simulink subsystem "ProcNav"  (R2021a)
settings: Solver=VariableStepAuto  StartTime=0.0  StopTime=10.0  RelTol=1e-3
undefined symbols (not defined in the file): DiscIntNeverNeededParam, physics
libraries: aerolibutil x9, sharedtransform x2, sharedTrackingLibrary x1
settings Model: Creator=Lamarre  LastModifiedBy=lamarre
settings SolverCC: AlgebraicLoopSolver=TrustRegion
settings DebuggingCC: SFMachineParentedDataDiag=warning

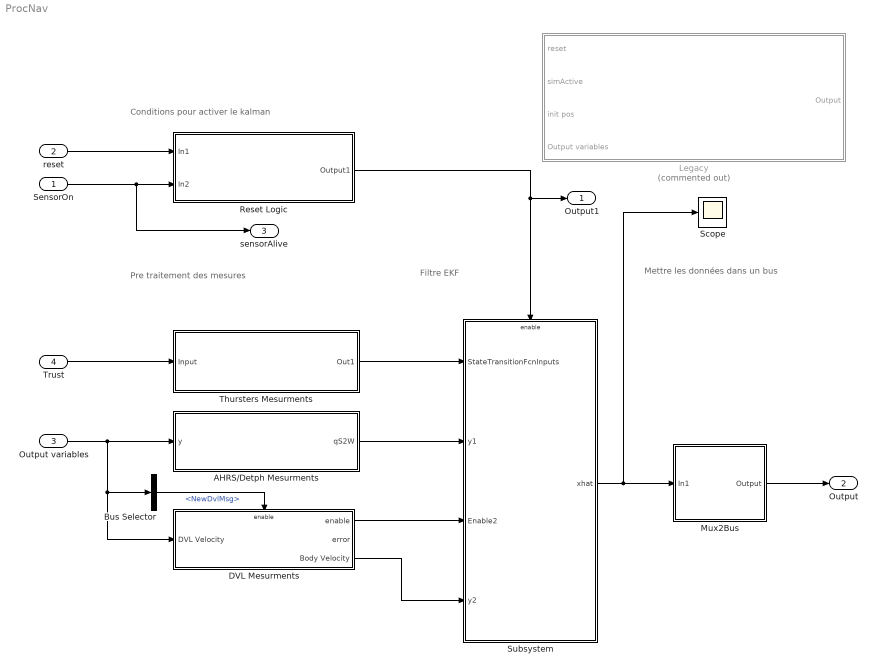
== system ProcNav ==
  note: Conditions pour activer le kalman
  note: Filtre EKF
  note: Pre traitement des mesures
  note: Mettre les données
      | dans un bus
  SensorOn : Inport
  reset : Inport  Port=2
  Output variables : Inport  Port=3
  Trust : Inport  Port=4
  AHRS/Detph Mesurments : Subsystem
  Bus Selector : BusSelector  OutputSignals=NewDvlMsg
  DVL Mesurments : Subsystem
  Legacy : Subsystem  Commented=on
  Mux2Bus : Subsystem
  Reset Logic : Subsystem
  Scope : Scope
  Subsystem : Subsystem
  Thursters Mesurments : Subsystem
  Output1 : Outport
  Output : Outport  Port=2
  sensorAlive : Outport  Port=3
  wires:
  DVL Mesurments/3(Body Velocity) -> Subsystem/4(y2)
  AHRS/Detph Mesurments/1(qS2W) -> Subsystem/2(y1)
  DVL Mesurments/1(enable) -> Subsystem/3(Enable2)
  Subsystem/1(xhat) -> Mux2Bus/1(In1), Scope/1
  Thursters Mesurments/1(Out1) -> Subsystem/1(StateTransitionFcnInputs)
  Output variables/1 -> DVL Mesurments/1(DVL Velocity), Bus Selector/1, AHRS/Detph Mesurments/1(y)
  Trust/1 -> Thursters Mesurments/1(Input)
  reset/1 -> Reset Logic/1(In1)
  SensorOn/1 -> Reset Logic/2(In2), sensorAlive/1
  Mux2Bus/1(Output) -> Output/1
  Bus Selector/1 -> DVL Mesurments/Enable  "<NewDvlMsg>"
  Reset Logic/1(Output1) -> Subsystem/Enable, Output1/1

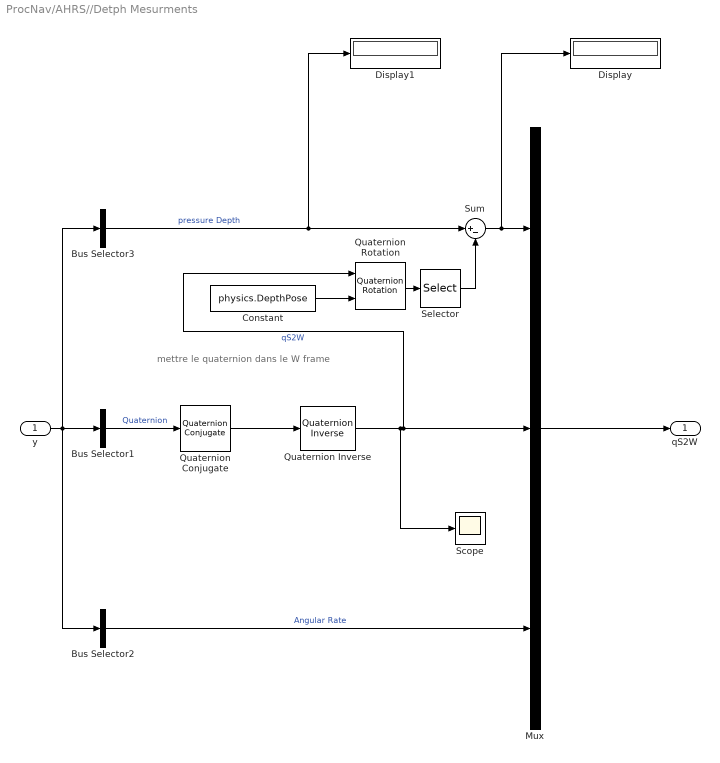
== system ProcNav/AHRS//Detph Mesurments ==
  note: mettre le quaternion dans le W frame
  y : Inport
  Bus Selector1 : BusSelector  OutputSignals=Quaternion  OutputAsBus=on
  Bus Selector2 : BusSelector  OutputSignals=Angular Rate  OutputAsBus=on
  Bus Selector3 : BusSelector  OutputSignals=Pressure Depth.Data  OutputAsBus=on
  Constant : Constant  Value=physics.DepthPose
  Display : Display
  Display1 : Display
  Mux : Mux  Inputs=3
  Quaternion Conjugate : aerolibutil/Quaternion Conjugate
      settings: SourceProductBaseCode=AE
  Quaternion Inverse : aerolibutil/Quaternion Inverse
  Quaternion Rotation : aerolibutil/Quaternion Rotation
  Scope : Scope
  Selector : Selector  InputPortWidth=3  IndexOptions=Index vector (dialog)  Indices=[3]  OutputSizes=1
  Sum : Sum  Inputs=|+-
  qS2W : Outport
  wires:
  Sum/1 -> Mux/1, Display/1
  Quaternion Rotation/1 -> Selector/1
  Selector/1 -> Sum/2
  Constant/1 -> Quaternion Rotation/2
  Bus Selector3/1 -> Sum/1, Display1/1  "pressure Depth"
  Quaternion Conjugate/1 -> Quaternion Inverse/1
  Mux/1 -> qS2W/1
  Bus Selector2/1 -> Mux/3  "Angular Rate"
  Quaternion Inverse/1 -> Mux/2, Quaternion Rotation/1, Scope/1  "qS2W"
  Bus Selector1/1 -> Quaternion Conjugate/1  "Quaternion"
  y/1 -> Bus Selector1/1, Bus Selector3/1, Bus Selector2/1

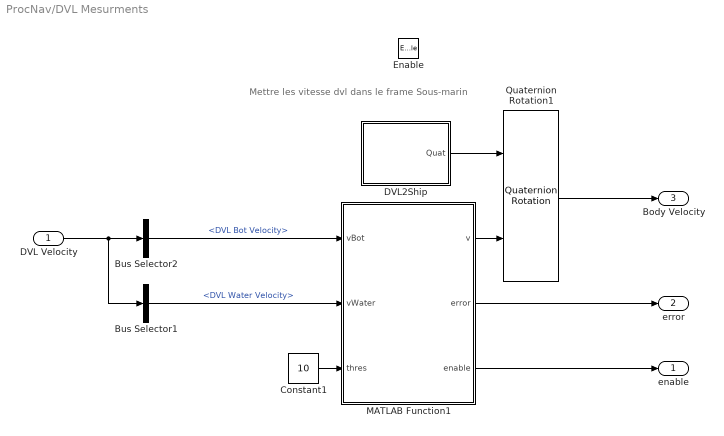
== system ProcNav/DVL Mesurments ==
  note: Mettre les vitesse dvl dans le frame Sous-marin
  DVL Velocity : Inport
  Enable : EnablePort
  Bus Selector1 : BusSelector  OutputSignals=DVL Water Velocity
  Bus Selector2 : BusSelector  OutputSignals=DVL Bot Velocity
  Constant1 : Constant  Value=10
  DVL2Ship : Subsystem
  MATLAB Function1 : MATLAB Function  TreatAsAtomicUnit=on
  Quaternion Rotation1 : aerolibutil/Quaternion Rotation
  enable : Outport
  error : Outport  Port=2
  Body Velocity : Outport  Port=3
  wires:
  MATLAB Function1/3(enable) -> enable/1
  Quaternion Rotation1/1 -> Body Velocity/1
  MATLAB Function1/2(error) -> error/1
  Bus Selector1/1 -> MATLAB Function1/2(vWater)  "<DVL Water Velocity>"
  Bus Selector2/1 -> MATLAB Function1/1(vBot)  "<DVL Bot Velocity>"
  DVL Velocity/1 -> Bus Selector2/1, Bus Selector1/1
  MATLAB Function1/1(v) -> Quaternion Rotation1/2
  Constant1/1 -> MATLAB Function1/3(thres)
  DVL2Ship/1(Quat) -> Quaternion Rotation1/1

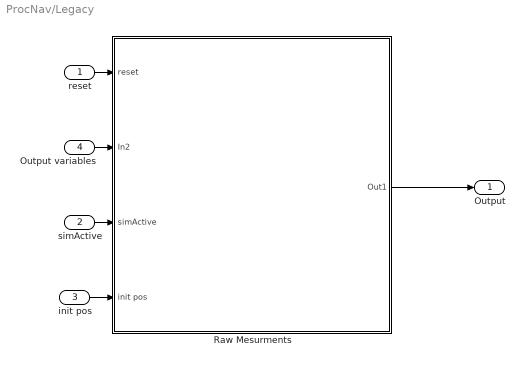
== system ProcNav/Legacy ==
  reset : Inport
  simActive : Inport  Port=2
  init pos : Inport  Port=3
  Output variables : Inport  Port=4
  "Raw Mesurments " : Subsystem
  Output : Outport
  wires:
  "Raw Mesurments "/1(Out1) -> Output/1
  init pos/1 -> "Raw Mesurments "/4(init pos)
  Output variables/1 -> "Raw Mesurments "/2(In2)
  reset/1 -> "Raw Mesurments "/1(reset)
  simActive/1 -> "Raw Mesurments "/3(simActive)

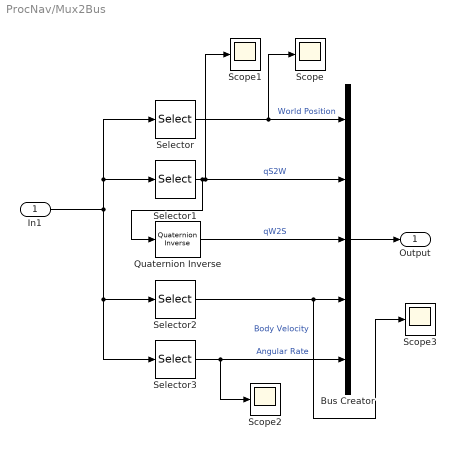
== system ProcNav/Mux2Bus ==
  In1 : Inport
  Bus Creator : BusCreator  Inputs=5
  Quaternion Inverse : aerolibutil/Quaternion Inverse
  Scope{,1..3} (4 alike) : Scope
  Selector : Selector  InputPortWidth=13  IndexOptions=Index vector (dialog)  Indices=[1:3]  OutputSizes=1
  Selector1 : Selector  InputPortWidth=13  IndexOptions=Index vector (dialog)  Indices=[4:7]  OutputSizes=1
  Selector2 : Selector  InputPortWidth=13  IndexOptions=Index vector (dialog)  Indices=[8:10]  OutputSizes=1
  Selector3 : Selector  InputPortWidth=13  IndexOptions=Index vector (dialog)  Indices=[11:13]  OutputSizes=1
  Output : Outport
  wires:
  Quaternion Inverse/1 -> Bus Creator/3  "qW2S"
  Selector2/1 -> Bus Creator/4, Scope3/1  "Body Velocity"
  Selector3/1 -> Bus Creator/5, Scope2/1  "Angular Rate"
  In1/1 -> Selector/1, Selector1/1, Selector2/1, Selector3/1
  Selector/1 -> Bus Creator/1, Scope/1  "World Position"
  Selector1/1 -> Bus Creator/2, Scope1/1, Quaternion Inverse/1  "qS2W"
  Bus Creator/1 -> Output/1

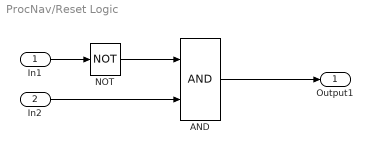
== system ProcNav/Reset Logic ==
  In1 : Inport
  In2 : Inport  Port=2
  AND : Logic  AllPortsSameDT=off  OutDataTypeStr=boolean
  NOT : Logic  Operator=NOT  AllPortsSameDT=off  OutDataTypeStr=boolean
  Output1 : Outport
  wires:
  AND/1 -> Output1/1
  In1/1 -> NOT/1
  NOT/1 -> AND/1
  In2/1 -> AND/2

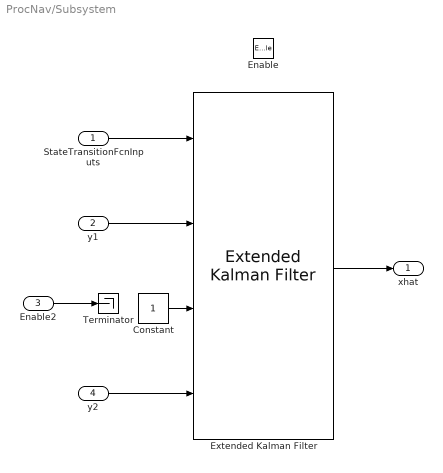
== system ProcNav/Subsystem ==
  StateTransitionFcnInputs : Inport
  y1 : Inport  Port=2
  Enable2 : Inport  Port=3
  y2 : Inport  Port=4
  Enable : EnablePort  StatesWhenEnabling=reset
  Constant : Constant
  Extended Kalman Filter : sharedTrackingLibrary/Extended Kalman Filter  StateTransitionFcn=EkfNavStatesEq  HasStateTransitionJacobianFcn=off  StateTransitionJacobianFcn=EkfNavJacobian  HasAdditiveProcessNoise=Additive  ProcessNoise=100  HasTimeVaryingProcessNoise=off  HasStateTransitionFcnExtraArgument=1  InitialState=[0,0,0.3,1,0,0,0,0,0,0,0,0,0]  InitialStateCovariance=[1,1,1,1,1,1,1,1,1,1,1,1,1]  MeasurementFcn1=EkfNavAhrsDepth  HasMeasurementJacobianFcn1=off  MeasurementJacobianFcn1=EkfJacobianNavAhrsDepth  HasMeasurementEnablePort1=off  HasAdditiveMeasurementNoise1=Additive  MeasurementNoise1=ones(1,8)*.1  HasTimeVaryingMeasurementNoise1=off  HasMeasurementFcnExtraArgument1=0  MeasurementFcn2=EkfNavDvl  HasMeasurementJacobianFcn2=off  MeasurementJacobianFcn2=EkfJacobianNavDvl  HasMeasurementEnablePort2=on  HasAdditiveMeasurementNoise2=Additive  MeasurementNoise2=ones(1,3)*0.1  HasTimeVaryingMeasurementNoise2=off  HasMeasurementFcnExtraArgument2=0  MeasurementFcn3=myMeasurementFcn  HasMeasurementJacobianFcn3=off  HasMeasurementEnablePort3=off  HasAdditiveMeasurementNoise3=Additive  MeasurementNoise3=1  HasTimeVaryingMeasurementNoise3=off  HasMeasurementFcnExtraArgument3=0  MeasurementFcn4=myMeasurementFcn  HasMeasurementJacobianFcn4=off  HasMeasurementEnablePort4=off  HasAdditiveMeasurementNoise4=Additive  MeasurementNoise4=1  HasTimeVaryingMeasurementNoise4=off  HasMeasurementFcnExtraArgument4=0  MeasurementFcn5=myMeasurementFcn  HasMeasurementJacobianFcn5=off  HasMeasurementEnablePort5=off  HasAdditiveMeasurementNoise5=Additive  MeasurementNoise5=1  HasTimeVaryingMeasurementNoise5=off  HasMeasurementFcnExtraArgument5=0  EnableMultirate=off  StateTransitionFcnSampleTime=1/20  MeasurementFcn1SampleTime=1/20  MeasurementFcn2SampleTime=1/10  MeasurementFcn3SampleTime=1  MeasurementFcn4SampleTime=1  MeasurementFcn5SampleTime=1  UseCurrentEstimator=on  OutputStateCovariance=off  DataType=double  SampleTime=1/20  NumberOfMeasurements=2
      settings: SourceProductBaseCode=CT,DR,TF,ID,LP,NV,AR,RO,RR,UV,VE
  Terminator : Terminator
  xhat : Outport
  wires:
  Enable2/1 -> Terminator/1
  Constant/1 -> Extended Kalman Filter/3
  y2/1 -> Extended Kalman Filter/4
  y1/1 -> Extended Kalman Filter/2
  StateTransitionFcnInputs/1 -> Extended Kalman Filter/1
  Extended Kalman Filter/1 -> xhat/1

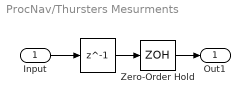
== system ProcNav/Thursters Mesurments ==
  Input : Inport
  " " : Delay  DelayLength=1  InitialCondition=[0,0,0,0,0,0,0,0]
  Zero-Order Hold : ZeroOrderHold  SampleTime=1/20
  Out1 : Outport
  wires:
  " "/1 -> Zero-Order Hold/1
  Zero-Order Hold/1 -> Out1/1
  Input/1 -> " "/1

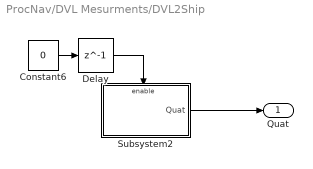
== system ProcNav/DVL Mesurments/DVL2Ship ==
  Constant6 : Constant  Value=0
  Delay : Delay  DelayLength=1  InitialCondition=1
  Subsystem2 : Subsystem
  Quat : Outport
  wires:
  Delay/1 -> Subsystem2/Enable
  Constant6/1 -> Delay/1
  Subsystem2/1(Quat) -> Quat/1

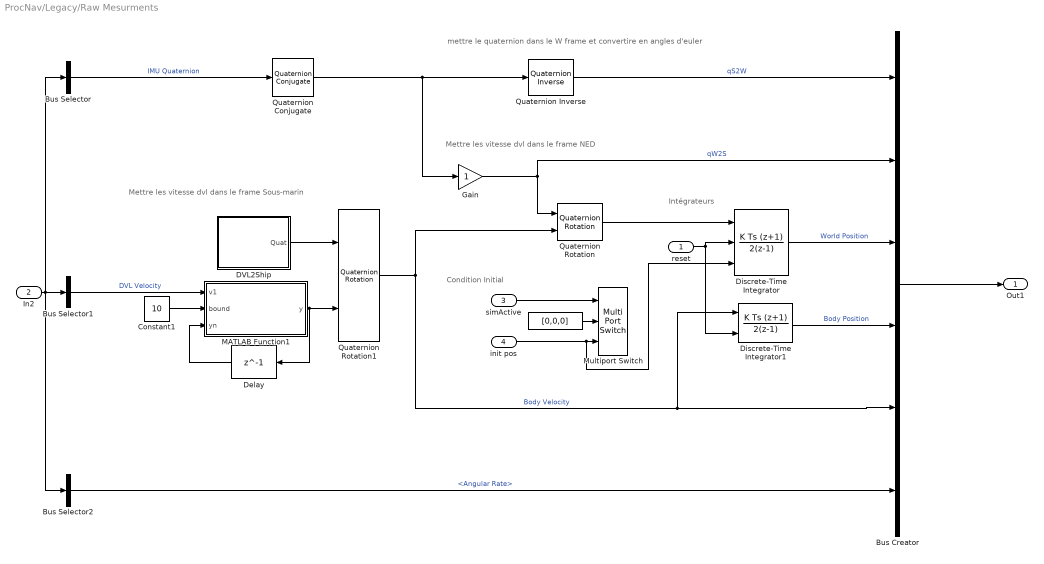
== system ProcNav/Legacy/Raw Mesurments  ==
  note: Mettre les vitesse dvl dans le frame Sous-marin
  note: Mettre les vitesse dvl dans le frame NED
  note: mettre le quaternion dans le W frame et convertire en angles d'euler
  note: Intégrateurs
  note: Condition Initial
  reset : Inport
  In2 : Inport  Port=2
  simActive : Inport  Port=3
  init pos : Inport  Port=4
  " " : Constant  Value=[0,0,0]
  Bus Creator : BusCreator  Inputs=6
  Bus Selector : BusSelector  OutputSignals=Quaternion  OutputAsBus=on
  Bus Selector1 : BusSelector  OutputSignals=DVL Bot Velocity  OutputAsBus=on
  Bus Selector2 : BusSelector  OutputSignals=Angular Rate
  Constant1 : Constant  Value=10
  DVL2Ship : Subsystem
  Delay : Delay  DelayLength=1  InitialCondition=0  UseCircularBuffer=on
  Discrete-Time Integrator : DiscreteIntegrator  IntegratorMethod=Integration: Trapezoidal  gainval=1%47/70  ExternalReset=rising  InitialConditionSource=external  SampleTime=1/20  ICPrevOutput=DiscIntNeverNeededParam  ICPrevScaledInput=DiscIntNeverNeededParam
  Discrete-Time Integrator1 : DiscreteIntegrator  IntegratorMethod=Integration: Trapezoidal  ExternalReset=rising  SampleTime=1/20  ICPrevOutput=DiscIntNeverNeededParam  ICPrevScaledInput=DiscIntNeverNeededParam
  Gain : Gain
  MATLAB Function1 : MATLAB Function  TreatAsAtomicUnit=on
  Multiport Switch : MultiPortSwitch  DataPortOrder=Zero-based contiguous  Inputs=2  zeroidx=on
  Quaternion Conjugate : aerolibutil/Quaternion Conjugate
      settings: SourceProductBaseCode=AE
  Quaternion Inverse : aerolibutil/Quaternion Inverse
  Quaternion Rotation : aerolibutil/Quaternion Rotation
  Quaternion Rotation1 : aerolibutil/Quaternion Rotation
  Out1 : Outport
  wires:
  Bus Selector2/1 -> Bus Creator/6  "<Angular Rate>"
  Discrete-Time Integrator1/1 -> Bus Creator/4  "Body Position"
  Bus Selector1/1 -> MATLAB Function1/1(v1)  "DVL Velocity"
  reset/1 -> Discrete-Time Integrator/2, Discrete-Time Integrator1/2
  Quaternion Rotation1/1 -> Quaternion Rotation/2, Discrete-Time Integrator1/1, Bus Creator/5  "Body Velocity"
  Bus Selector/1 -> Quaternion Conjugate/1  "IMU Quaternion"
  Delay/1 -> MATLAB Function1/3(yn)
  " "/1 -> Multiport Switch/2
  Gain/1 -> Bus Creator/2, Quaternion Rotation/1  "qW2S"
  Bus Creator/1 -> Out1/1
  simActive/1 -> Multiport Switch/1
  MATLAB Function1/1(y) -> Quaternion Rotation1/2, Delay/1
  In2/1 -> Bus Selector1/1, Bus Selector/1, Bus Selector2/1
  Quaternion Conjugate/1 -> Quaternion Inverse/1, Gain/1
  init pos/1 -> Multiport Switch/3, Discrete-Time Integrator/3
  Quaternion Inverse/1 -> Bus Creator/1  "qS2W"
  Constant1/1 -> MATLAB Function1/2(bound)
  Quaternion Rotation/1 -> Discrete-Time Integrator/1
  DVL2Ship/1(Quat) -> Quaternion Rotation1/1
  Discrete-Time Integrator/1 -> Bus Creator/3  "World Position"

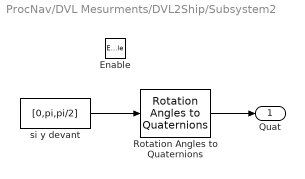
== system ProcNav/DVL Mesurments/DVL2Ship/Subsystem2 ==
  Enable : EnablePort
  Rotation Angles to Quaternions : sharedtransform/Rotation Angles to Quaternions  rotationOrder=XYZ  aMode=aMode
      settings: SourceProductBaseCode=AE,PW,MT,VE,VP
  si y devant : Constant  Value=[0,pi,pi/2]
  Quat : Outport
  wires:
  Rotation Angles to Quaternions/1 -> Quat/1
  si y devant/1 -> Rotation Angles to Quaternions/1

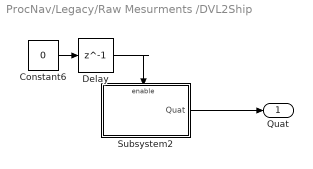
== system ProcNav/Legacy/Raw Mesurments /DVL2Ship ==
  Constant6 : Constant  Value=0
  Delay : Delay  DelayLength=1  InitialCondition=1
  Subsystem2 : Subsystem
  Quat : Outport
  wires:
  Delay/1 -> Subsystem2/Enable
  Constant6/1 -> Delay/1
  Subsystem2/1(Quat) -> Quat/1

== system ProcNav/Legacy/Raw Mesurments /DVL2Ship/Subsystem2 ==
  Enable : EnablePort
  Rotation Angles to Quaternions : sharedtransform/Rotation Angles to Quaternions  rotationOrder=XYZ  aMode=aMode
      settings: SourceProductBaseCode=AE,PW,MT,VE,VP
  si y devant : Constant  Value=[0,pi,pi/2]
  Quat : Outport
  wires:
  Rotation Angles to Quaternions/1 -> Quat/1
  si y devant/1 -> Rotation Angles to Quaternions/1

== matlab function ProcNav/Legacy/Raw Mesurments /MATLAB Function1 ==
  data: v1 input; y output; bound input; yn input
function y = DVLWrap(v1,bound,yn)

 for i=1: size(v1,1)
     if v1(i)<-bound || v1(i)>bound
         v1(i)=yn(i);
     end
 end
y = v1(1:3);

== matlab function ProcNav/DVL Mesurments/MATLAB Function1 ==
  data: vBot input; vWater input; v output; error output; thres input; enable output
function [v, error, enable] = DVLManager(vBot,vWater,thres)

    if max(abs(vBot))< thres
        %retouner les vitesse du bottom tracking (normal)
        v = vBot(1:3);
        enable = 1;
        error = ones(1,3) * vBot(4);
    elseif max(abs(vWater))< thres
        % retouner les vitesse du water profiling si bottom tracking fail
        v = vWater(1:3);
        enable = 0;
        error = ones(1,3) * vWater(4);
    else
        % Désactiver le dvl si mauvais data
        v = zeros(3,1);
        enable = 0;
        error = ones(1,3) * vBot(4);
    end
end
